simulink model "ex8_2"  (R2021b)
settings: Solver=VariableStepAuto  StartTime=0.0  StopTime=4  FixedStep=1e-4  EnableMultiTasking=on
settings Model: Creator=user  LastModifiedBy=chesterXalan
settings SolverCC: AlgebraicLoopSolver=TrustRegion
settings DataIOCC: LimitDataPoints=on  ReturnWorkspaceOutputs=off
settings OptimizationCC: LifeSpan=inf
settings DebuggingCC: AllowSymbolicDim=off  SFUnexpectedBacktrackingDiag=warning  SFNoUnconditionalDefaultTransitionDiag=warning  SFExecutionAtInitializationDiag=none  SFMachineParentedDataDiag=warning  ArithmeticOperatorsInVariantConditions=warning
settings ModelReferenceCC: PropagateSignalLabelsOutOfModel=off
settings SFSimCC: SimUseLocalCustomCode=off  CustomCodeUndefinedFunction=UseInterfaceOnly
settings RTWCC: RTWUseLocalCustomCode=off
settings CodeAppCC: StateflowObjectComments=on
settings GRTTargetCC: TargetLangStandard=C89/C90 (ANSI)
settings ConfigComp: CovMetricSettings=dw  CovSaveCumulativeToWorkspaceVar=on  CovSaveSingleToWorkspaceVar=on  CovExternalEMLEnable=off

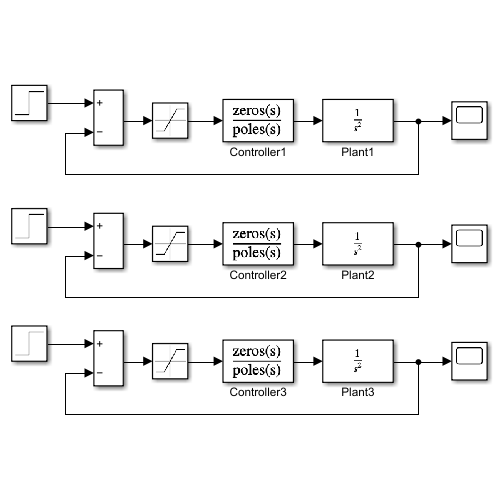
[thumbnail: Simulink's stored preview of the top-level diagram]
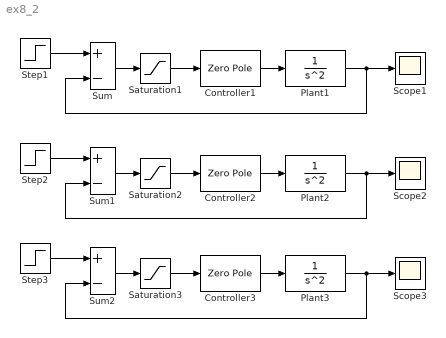
== system ex8_2 ==
  Controller1 : ZeroPole  Zeros=[-1]  Poles=[-5]  Gain=[10]
  Controller2 : ZeroPole  Zeros=[-1]  Poles=[-3]  Gain=[8]
  Controller3 : ZeroPole  Zeros=[-1]  Poles=[-5]  Gain=[50]
  Plant1 : TransferFcn  Denominator=[1 0 0]
  Plant2 : TransferFcn  Denominator=[1 0 0]
  Plant3 : TransferFcn  Denominator=[1 0 0]
  Saturation1 : Saturate  UpperLimit=1  LowerLimit=-1
  Saturation2 : Saturate  UpperLimit=1  LowerLimit=-1
  Saturation3 : Saturate  UpperLimit=1  LowerLimit=-1
  Scope1 : Scope
  Scope2 : Scope
  Scope3 : Scope
  Step1 : Step  Time=0.01  SampleTime=1e-3
  Step2 : Step  Time=0.01  SampleTime=1e-3
  Step3 : Step  Time=0.01  SampleTime=1e-3
  Sum : Sum  Inputs=+-
  Sum1 : Sum  Inputs=+-
  Sum2 : Sum  Inputs=+-
  wires:
  Step1/1 -> Sum/1
  Controller1/1 -> Plant1/1
  Plant1/1 -> Sum/2, Scope1/1
  Sum/1 -> Saturation1/1
  Saturation1/1 -> Controller1/1
  Step2/1 -> Sum1/1
  Controller2/1 -> Plant2/1
  Plant2/1 -> Sum1/2, Scope2/1
  Sum1/1 -> Saturation2/1
  Saturation2/1 -> Controller2/1
  Step3/1 -> Sum2/1
  Controller3/1 -> Plant3/1
  Plant3/1 -> Sum2/2, Scope3/1
  Sum2/1 -> Saturation3/1
  Saturation3/1 -> Controller3/1
